simulink model "cw8_model_P_PI_PID_Relidzynski"  (R2022a)
settings: Solver=VariableStepAuto  StartTime=0.0  StopTime=200.0  MaxStep=0.01  MinStep=0.001  RelTol=1e-6
values from neighbouring files (symbols this model uses):
  A = [-1/(R1*C1), 1/(R1*C1), 0 ... (first row only)    [cw8_dane_Relidzynski.m]
  B = [1/C1;0;0]    [cw8_dane_Relidzynski.m]
  C = [0,0,1]    [cw8_dane_Relidzynski.m]
  D = [0]    [cw8_dane_Relidzynski.m]
  k = 100    [cw8_dane_Relidzynski.m]
  P0 = 1    [cw8_dane_Relidzynski.m]
settings Model: Creator=User  LastModifiedBy=Radosław
settings SolverCC: AlgebraicLoopSolver=TrustRegion
settings DataIOCC: SaveFormat=Array  ReturnWorkspaceOutputs=off
settings DebuggingCC: UnconnectedInputMsg=warning  UnconnectedOutputMsg=warning  UnconnectedLineMsg=warning  SFMachineParentedDataDiag=warning  ArithmeticOperatorsInVariantConditions=warning
settings SFSimCC: SimUseLocalCustomCode=off  CustomCodeUndefinedFunction=UseInterfaceOnly
settings RTWCC: RTWUseLocalCustomCode=off

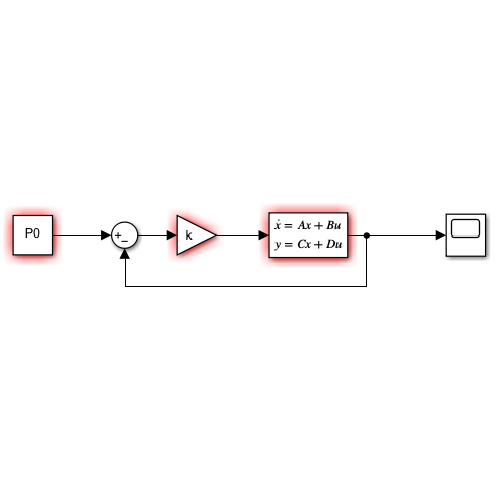
[thumbnail: Simulink's stored preview of the top-level diagram]
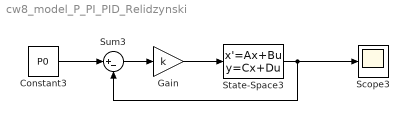
== system cw8_model_P_PI_PID_Relidzynski ==
  Constant3 : Constant  Value=P0
  Gain : Gain  Gain=k
  Scope3 : Scope
  State-Space3 : StateSpace  A=A  B=B  C=C  D=D  InitialCondition=0
  Sum3 : Sum  Inputs=|+-
  wires:
  Sum3/1 -> Gain/1
  State-Space3/1 -> Scope3/1, Sum3/2
  Gain/1 -> State-Space3/1
  Constant3/1 -> Sum3/1
